simulink model "Buck_Converter"  (R2015b)
settings: Solver=VariableStepAuto  StartTime=0.0  StopTime=0.01  RelTol=1e-3
values from neighbouring files (symbols this model uses):
  controller_on = true    [parameters.m]
  current_sense = 0.02    [parameters.m]
  D = 0.4    [parameters.m]
  G_II_C = 0    [parameters.m]
  G_II_L = 0    [parameters.m]
  Rload = R_saved    [ToleranzSimulation.m]    (also in parameters.m = 10000)
  T = T_saved    [ToleranzSimulation.m]    (also in parameters.m = 1.25e-05)
  Uin = 200    [parameters.m]
  Uswitch = 5    [parameters.m]
libraries: fl_lib x17, nesl_utility x10, elec_lib x3
settings Model: Creator=lukaskiechle  LastModifiedBy=lukaskiechle
settings DebuggingCC: MaxConsecutiveZCsMsg=none
settings SimscapeCC: SimscapeLogType=all

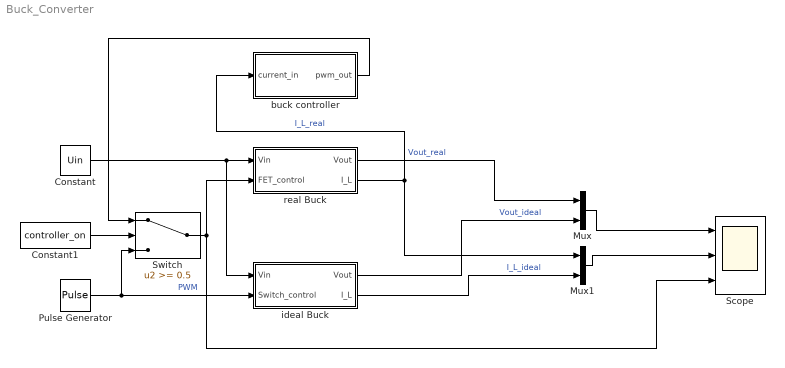
== system Buck_Converter ==
  Constant : Constant  Value=Uin
  Constant1 : Constant  Value=controller_on
  Mux : Mux  Inputs=2
      settings: DisplayOption=signals
  Mux1 : Mux  Inputs=2
      settings: DisplayOption=signals
  Pulse Generator : DiscretePulseGenerator  PulseType=Time based  Amplitude=Uswitch  Period=T  PulseWidth=D*100  PhaseDelay=T
  Scope : Scope  NumInputPorts=3
  Switch : Switch  Threshold=0.5
  buck controller : Subsystem
  ideal Buck : Subsystem
  real Buck : Subsystem
  wires:
  Constant/1 -> ideal Buck/1(Vin), real Buck/1(Vin)
  real Buck/1(Vout) -> Mux/1  "Vout_real"
  real Buck/2(I_L) -> Mux1/1, buck controller/1(current_in)  "I_L_real"
  ideal Buck/1(" Vout") -> Mux/2  "Vout_ideal"
  ideal Buck/2(I_L) -> Mux1/2  "I_L_ideal"
  Mux1/1 -> Scope/2
  Mux/1 -> Scope/1
  Switch/1 -> Scope/3, real Buck/2(FET_control)
  Pulse Generator/1 -> ideal Buck/2(Switch_control), Switch/3  "PWM"
  Constant1/1 -> Switch/2
  buck controller/1(pwm_out) -> Switch/1

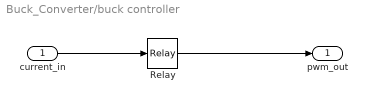
== system Buck_Converter/buck controller ==
  current_in : Inport
  Relay : Relay  OnSwitchValue=current_sense  OffSwitchValue=0  OnOutputValue=0  OffOutputValue=Uswitch
  pwm_out : Outport
  wires:
  current_in/1 -> Relay/1
  Relay/1 -> pwm_out/1

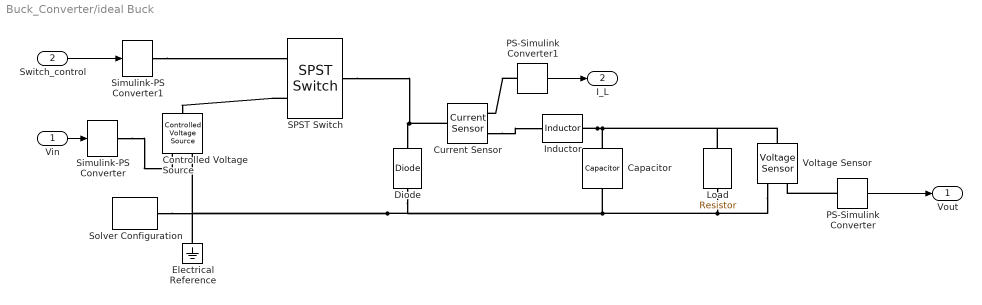
== system Buck_Converter/ideal Buck ==
  Vin : Inport
  Switch_control : Inport  Port=2
  Capacitor : fl_lib/Electrical/Electrical Elements/Capacitor  c=C F  r=0.0001 Ohm  g=0 1/Ohm  i_specify=off  i_priority=None  i=0 A  v_specify=off  v_priority=None  v=0 V  vc_specify=off  vc_priority=None  vc=0 V
  Controlled Voltage Source : fl_lib/Electrical/Electrical Sources/Controlled Voltage Source
  Current Sensor : fl_lib/Electrical/Electrical Sensors/Current Sensor
  Diode : fl_lib/Electrical/Electrical Elements/Diode  Vf=0.7 V  Ron=0.0001 Ohm  Goff=1e-9 1/Ohm  i_specify=off  i_priority=None  i=0 A  v_specify=off  v_priority=None  v=0 V
  Electrical Reference : fl_lib/Electrical/Electrical Elements/Electrical Reference
  Inductor : fl_lib/Electrical/Electrical Elements/Inductor  l=L H  r=0.0001 Ohm  g=0 1/Ohm  i_specify=off  i_priority=None  i=0 A  v_specify=off  v_priority=None  v=0 V  i_L_specify=off  i_L_priority=None  i_L=0 A
  Load : fl_lib/Electrical/Electrical Elements/Resistor  R=Rload Ohm  i_specify=off  i_priority=None  i=0 A  v_specify=off  v_priority=None  v=0 V
  PS-Simulink Converter : nesl_utility/PS-Simulink Converter  PhysicalDomain=network_engine_domain  SubClassName=ps_output  LeftPortType=input  RightPortType=output  PseudoPeriodic=off  Frequencies=[]  Unit=V  AffineConversion=off
  PS-Simulink Converter1 : nesl_utility/PS-Simulink Converter  PhysicalDomain=network_engine_domain  SubClassName=ps_output  LeftPortType=input  RightPortType=output  PseudoPeriodic=off  Frequencies=[]  Unit=A  AffineConversion=off
  SPST Switch : elec_lib/Passive Devices/Switches/SPST Switch  R_closed=0.0001 Ohm  G_open=1e-6 S  Threshold=0.5 V  Width=0 V  model_dynamics=0  t_on=0.001 s  t_off=0.001 s  initial_vT=0 V
  Simulink-PS Converter : nesl_utility/Simulink-PS Converter  PhysicalDomain=network_engine_domain  SubClassName=ps_input  LeftPortType=input  RightPortType=output  PseudoPeriodic=off  Frequencies=[]  NoiseDistribution=none  NoiseParameters=[]  Unit=1  AffineConversion=off  InputFiltering=off  SimscapeFilterOrder=1  InputFilterTimeConstant=0.001  UdotUserProvided=1
  Simulink-PS Converter1 : nesl_utility/Simulink-PS Converter  PhysicalDomain=network_engine_domain  SubClassName=ps_input  LeftPortType=input  RightPortType=output  PseudoPeriodic=off  Frequencies=[]  NoiseDistribution=none  NoiseParameters=[]  Unit=V  AffineConversion=off  InputFiltering=off  SimscapeFilterOrder=1  InputFilterTimeConstant=0.001  UdotUserProvided=1
  Solver Configuration : nesl_utility/Solver Configuration  PhysicalDomain=network_engine_domain  SubClassName=solver  LeftPortType=input  RightPortType=generic  Accelerate=off  Tones=[]  Harmonics=[]  SimulateNoise=off  Profile=off  UseLocalSampling=off  EnableSwitchedLinearOptims=on  FrequencyDomain=off  UseCCode=off  RelTol=0.001  AbsTol=1e-06  MinStep=1e-09  ToWorkspace=off  RevertToSquareIcSolve=off  NumHomotopyIterations=100  PhasorMode=off  PhasorModeNumHarmonics=1  DoDC=on  ResidualTolerance=1e-09  UseLocalSolver=off  LocalSolverChoice=NE_BACKWARD_EULER_ADVANCER  LocalSolverSampleTime=0.001  DoFixedCost=off  MaxNonlinIter=3  MaxModeIter=2  LinearAlgebra=Sparse  DelaysMemoryBudget=1024  AutomaticFiltering=on  FilteringTimeConstant=0.001
  Voltage Sensor : fl_lib/Electrical/Electrical Sensors/Voltage Sensor
  " Vout" : Outport
  I_L : Outport  Port=2
  wires:
  PS-Simulink Converter/1 -> " Vout"/1
  Vin/1 -> Simulink-PS Converter/1
  PS-Simulink Converter1/1 -> I_L/1
  Switch_control/1 -> Simulink-PS Converter1/1
  connections:
  Current Sensor/LConn1 -- SPST Switch/RConn1 -- Diode/RConn1
  Inductor/RConn1 -- Capacitor/LConn1 -- Voltage Sensor/LConn1 -- Load/LConn1
  Voltage Sensor/RConn2 -- Load/RConn1 -- Diode/LConn1 -- Controlled Voltage Source/RConn2 -- Solver Configuration/RConn1 -- Electrical Reference/LConn1 -- Capacitor/RConn1
  PS-Simulink Converter/LConn1 -- Voltage Sensor/RConn1
  Current Sensor/RConn2 -- Inductor/LConn1
  Simulink-PS Converter/RConn1 -- Controlled Voltage Source/RConn1
  PS-Simulink Converter1/LConn1 -- Current Sensor/RConn1
  SPST Switch/LConn2 -- Controlled Voltage Source/LConn1
  Simulink-PS Converter1/RConn1 -- SPST Switch/LConn1

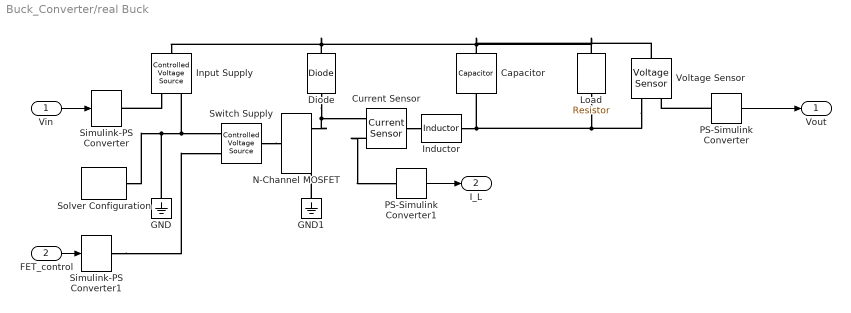
== system Buck_Converter/real Buck ==
  Vin : Inport
  FET_control : Inport  Port=2
  Capacitor : fl_lib/Electrical/Electrical Elements/Capacitor  c=C F  r=R_serie_C Ohm  g=G_II_C 1/Ohm  i_specify=off  i_priority=None  i=0 A  v_specify=off  v_priority=None  v=0 V  vc_specify=off  vc_priority=None  vc=0 V
  Current Sensor : fl_lib/Electrical/Electrical Sensors/Current Sensor
  Diode : elec_lib/Semiconductor Devices/Diode  ModelType=1  Vf=U_Diode V  Ron=R_on_Diode Ohm  Goff=G_off_Diode S  Rz=0.3 Ohm  Vz=500 V  C_PWL=C_Diode F  prmExp=1  I12=[ 0.0137 0.545 ] A  V12=[ 0.6 0.7 ] V  I1=0.0137 A  V1=0.6 V  RS=0.01 Ohm  IS=1e-12 A  Tmeas=25 C  ec=1  BV=Inf V  C_param=1  CJ0=5 pF  VJ=1 V  Mgrad=0.5  Vvec=[ 0.1 10 100 ] V  Cvec=[ 3.5 1 0.4 ] pF  FC=0.5  Q_param=1  Irrm=-7.15 A  iF=4 A  didt=-750 A/us  trr=115 ns  TT=50 ns  tau=100 ns  T_param=1  IS_T2=1.25e-7 A  I1_T2=0.245 A  V1_T2=0.5 V  Tmeas2=125 C  EG_param=1  EG=1.11 eV  XTI_param=1  XTI=3  dBVdT=0 V/K  Tdevice=25 C  Rth=[ 0 10 ] K/W  thermal_mass_parameterization=1  thermal_mass=[ 0 1 ] J/K  thermal_time_constant=[ 0 10 ] s  thermal_mass_initial_temperatures=[ 25 25 ] C
  GND : fl_lib/Electrical/Electrical Elements/Electrical Reference
  GND1 : fl_lib/Electrical/Electrical Elements/Electrical Reference
  Inductor : fl_lib/Electrical/Electrical Elements/Inductor  l=L H  r=R_serie_L Ohm  g=G_II_L 1/Ohm  i_specify=off  i_priority=None  i=0 A  v_specify=off  v_priority=None  v=0 V  i_L_specify=off  i_L_priority=None  i_L=0 A
  Input Supply : fl_lib/Electrical/Electrical Sources/Controlled Voltage Source
  Load : fl_lib/Electrical/Electrical Elements/Resistor  R=Rload Ohm  i_specify=off  i_priority=None  i=0 A  v_specify=off  v_priority=None  v=0 V
  N-Channel MOSFET : elec_lib/Semiconductor Devices/N-Channel MOSFET  parameterization=1  prmDatasheet=1  prmEquCoeff=1  Beta=5 A/V^2  Rds=R_DS_on Ohm  Id=Ids A  Vgs=Vgs V  Vth=Vth V  lam=0 1/V  Tmeas=25 C  RS=R_S_FET Ohm  RD=R_D_FET Ohm  C_param=1  C_GS=270 pF  C_GD=80 pF  C_iss=C_iss F  C_rss=C_rss F  C_oss=C_oss F  C_GS_vec=[ 270 300 290 280 295 255 ] pF  C_GD_vec=[ 450 400 300 190 95 55 ] pF  C_iss_vec=[ 720 700 590 470 390 310 ] pF  C_rss_vec=[ 450 400 300 190 95 55 ] pF  C_oss_vec=[ 900 810 690 420 270 170 ] pF  C_Vds_vec=[ 0.1 0.3 1 3 10 30 ] V  charge_linearity_param=1  C_OX=200 pF  V_C_OX=-0.5 V  dVth_dT=-6 mV/K  Rds_T2=0.037 Ohm  Tmeas2=125 C  BEXDatasheet=-1.5  BEXEquCoeff=-1.5  TdeviceDatasheet=25 C  TdeviceEquCoeff=25 C  Rth=[ 0 10 ] K/W  thermal_mass_parameterization=1  thermal_mass=[ 0 1 ] J/K  thermal_time_constant=[ 0 10 ] s  thermal_mass_initial_temperatures=[ 25 25 ] C
  PS-Simulink Converter : nesl_utility/PS-Simulink Converter  PhysicalDomain=network_engine_domain  SubClassName=ps_output  LeftPortType=input  RightPortType=output  PseudoPeriodic=off  Frequencies=[]  Unit=V  AffineConversion=off
  PS-Simulink Converter1 : nesl_utility/PS-Simulink Converter  PhysicalDomain=network_engine_domain  SubClassName=ps_output  LeftPortType=input  RightPortType=output  PseudoPeriodic=off  Frequencies=[]  Unit=A  AffineConversion=off
  Simulink-PS Converter : nesl_utility/Simulink-PS Converter  PhysicalDomain=network_engine_domain  SubClassName=ps_input  LeftPortType=input  RightPortType=output  PseudoPeriodic=off  Frequencies=[]  NoiseDistribution=none  NoiseParameters=[]  Unit=V  AffineConversion=off  InputFiltering=off  SimscapeFilterOrder=1  InputFilterTimeConstant=0.001  UdotUserProvided=1
  Simulink-PS Converter1 : nesl_utility/Simulink-PS Converter  PhysicalDomain=network_engine_domain  SubClassName=ps_input  LeftPortType=input  RightPortType=output  PseudoPeriodic=off  Frequencies=[]  NoiseDistribution=none  NoiseParameters=[]  Unit=V  AffineConversion=off  InputFiltering=off  SimscapeFilterOrder=1  InputFilterTimeConstant=0.001  UdotUserProvided=1
  Solver Configuration : nesl_utility/Solver Configuration  PhysicalDomain=network_engine_domain  SubClassName=solver  LeftPortType=input  RightPortType=generic  Accelerate=off  Tones=[]  Harmonics=[]  SimulateNoise=off  Profile=off  UseLocalSampling=off  EnableSwitchedLinearOptims=on  FrequencyDomain=off  UseCCode=off  RelTol=0.001  AbsTol=1e-06  MinStep=1e-09  ToWorkspace=off  RevertToSquareIcSolve=off  NumHomotopyIterations=100  PhasorMode=off  PhasorModeNumHarmonics=1  DoDC=on  ResidualTolerance=1e-09  UseLocalSolver=off  LocalSolverChoice=NE_BACKWARD_EULER_ADVANCER  LocalSolverSampleTime=0.001  DoFixedCost=off  MaxNonlinIter=3  MaxModeIter=2  LinearAlgebra=Sparse  DelaysMemoryBudget=1024  AutomaticFiltering=on  FilteringTimeConstant=0.001
  Switch Supply : fl_lib/Electrical/Electrical Sources/Controlled Voltage Source
  Voltage Sensor : fl_lib/Electrical/Electrical Sensors/Voltage Sensor
  Vout : Outport
  I_L : Outport  Port=2
  wires:
  PS-Simulink Converter/1 -> Vout/1
  Vin/1 -> Simulink-PS Converter/1
  FET_control/1 -> Simulink-PS Converter1/1
  PS-Simulink Converter1/1 -> I_L/1
  connections:
  Capacitor/LConn1 -- Voltage Sensor/LConn1 -- Load/LConn1 -- Input Supply/LConn1 -- Diode/RConn1
  Voltage Sensor/RConn2 -- Load/RConn1 -- Inductor/LConn1 -- Capacitor/RConn1
  N-Channel MOSFET/RConn1 -- Current Sensor/RConn2 -- Diode/LConn1
  Switch Supply/LConn1 -- N-Channel MOSFET/LConn1
  PS-Simulink Converter/LConn1 -- Voltage Sensor/RConn1
  GND1/LConn1 -- N-Channel MOSFET/RConn2
  GND/LConn1 -- Solver Configuration/RConn1 -- Switch Supply/RConn2 -- Input Supply/RConn2
  Input Supply/RConn1 -- Simulink-PS Converter/RConn1
  Simulink-PS Converter1/RConn1 -- Switch Supply/RConn1
  Current Sensor/LConn1 -- Inductor/RConn1
  Current Sensor/RConn1 -- PS-Simulink Converter1/LConn1
